simulink model "SASA_two_piezo"  (R2016a)
settings: Solver=FixedStepAuto  SolverMode=SingleTasking  StartTime=0.0  StopTime=200  FixedStep=1e-4  MaxStep=0.00001  MinStep=0.000000001  RelTol=1e-3  AbsTol=1e-3
values from neighbouring files (symbols this model uses):
  A = zeros(modes,modes)    [matrice_two_piezo.m]
  B = zeros(modes,modes)    [matrice_two_piezo.m]
  C = zeros(1,modes)    [matrice_two_piezo.m]
  c = c_num/c_den    (= -1.2195777478e-05)    [matrice_two_piezo.m]
  D = zeros(modes,modes)    [matrice_two_piezo.m]
  E = zeros(modes,modes)    [matrice_two_piezo.m]
  Q = double(Q)    [matrice_two_piezo.m]
settings Model: ExtModeTrigDuration=2  Creator=yashwanth  LastModifiedBy=yash9
settings DataIOCC: LimitDataPoints=on  SaveFormat=Array
settings OptimizationCC: OptimizeModelRefInitCode=on  MaxStackSize=64
settings DebuggingCC: SolverPrmCheckMsg=warning  AllowSymbolicDim=off
settings HardwareCC: ProdBitPerLong=64  ProdLargestAtomicFloat=None  ProdHWDeviceType=Intel->x86-64  TargetBitPerLong=64  TargetBitPerPointer=64  TargetIntDivRoundTo=Zero  TargetEndianess=LittleEndian  TargetWordSize=64  TargetHWDeviceType=Intel->x86-64
settings ModelReferenceCC: PropagateSignalLabelsOutOfModel=off
settings RTWCC: SystemTargetFile=sldrtert.tlc  TemplateMakefile=sldrtert.tmf  Description=Simulink Desktop Real-Time (ERT)  Toolchain=Arduino AVR v1.6.1  BuildConfiguration=Faster Runs  TargetLang=C++  RTWCompilerOptimization=on
settings CodeAppCC: IgnoreCustomStorageClasses=off  MaxIdLength=95
settings SimulinkDesktopRealTimeERTCC: TargetFcnLib=ansi_tfl_table_tmw.mat  TargetLibSuffix=_sldrt.lib  TargetPreCompLibLocation=C:\Program Files\MATLAB\R2016a\toolbox\sldrt\lib\win64  GenFloatMathFcnCalls=NOT IN USE  TargetLangStandard=C89/C90 (ANSI)  CodeReplacementLibrary=None  UtilityFuncGeneration=Auto  ERTMultiwordTypeDef=System defined  ERTMultiwordLength=256  MultiwordLength=2048  GenerateFullHeader=on  InferredTypesCompatibility=off  GenerateSampleERTMain=off  GenerateTestInterfaces=off  ModelReferenceCompliant=on  ParMdlRefBuildCompliant=off  CompOptLevelCompliant=on  ConcurrentExecutionCompliant=off  IncludeMdlTerminateFcn=on  GeneratePreprocessorConditionals=Use local settings  CombineOutputUpdateFcns=off  CombineSignalStateStructs=off  SuppressErrorStatus=off  ERTFirstTimeCompliant=off  IncludeFileDelimiter=Auto  ERTCustomFileBanners=off  SupportAbsoluteTime=on  LogVarNameModifier=rt_  MatFileLogging=off  MultiInstanceERTCode=off  CodeInterfacePackaging=Nonreusable function  SupportNonFinite=on  SupportComplex=on  PurelyIntegerCode=off  SupportContinuousTime=on  SupportNonInlinedSFcns=on  SupportVariableSizeSignals=off  ParenthesesLevel=Nominal  CastingMode=Nominal  MATLABClassNameForMDSCustomization=Simulink.SoftwareTarget.TargetSpecificTriggerConfigurationBase  ModelStepFunctionPrototypeControlCompliant=off  CPPClassGenCompliant=off  AutosarCompliant=off  GRTInterface=off  GenerateAllocFcn=off  UseToolchainInfoCompliant=off  GenerateSharedConstants=on  GenerateASAP2=off  InlinedParameterPlacement=Hierarchical  TargetOS=BareBoardExample  MultiInstanceErrorCode=Error  RateGroupingCode=on  RootIOFormat=Individual arguments  RTWCAPISignals=off  RTWCAPIParams=off  RTWCAPIStates=off  RTWCAPIRootIO=off  ERTSrcFileBannerTemplate=ert_code_template.cgt  ERTHdrFileBannerTemplate=ert_code_template.cgt  ERTDataSrcFileTemplate=ert_code_template.cgt  ERTDataHdrFileTemplate=ert_code_template.cgt  ERTCustomFileTemplate=example_file_process.tlc  EnableDataOwnership=off  SignalDisplayLevel=10  ParamTuneLevel=10  GlobalDataDefinition=Auto  DataDefinitionFile=global.c  GlobalDataReference=Auto  ERTFilePackagingFormat=Modular  DataReferenceFile=global.h  PreserveExpressionOrder=off  PreserveIfCondition=off  ConvertIfToSwitch=off  PreserveExternInFcnDecls=on  SuppressUnreachableDefaultCases=off  EnableSignedLeftShifts=on  EnableSignedRightShifts=on  IndentStyle=K&R  IndentSize=2  EnableUserReplacementTypes=off  MaxIdInt32=MAX_int32_T  MinIdInt32=MIN_int32_T  MaxIdUint32=MAX_uint32_T  MaxIdInt16=MAX_int16_T  MinIdInt16=MIN_int16_T  MaxIdUint16=MAX_uint16_T  MaxIdInt8=MAX_int8_T  MinIdInt8=MIN_int8_T  MaxIdUint8=MAX_uint8_T  BooleanTrueId=true  BooleanFalseId=false  MemSecPackage=--- None ---  MemSecDataConstants=Default  MemSecDataIO=Default  MemSecDataInternal=Default  MemSecDataParameters=Default  MemSecFuncInitTerm=Default  MemSecFuncExecute=Default  MemSecFuncSharedUtil=Default  CCListing=off  RebuildAll=off  ExtMode=on  ExtModeTransport=0  ExtModeStaticAlloc=off  ExtModeStaticAllocSize=1000000  ExtModeTesting=off  ExtModeMexFile=sldrtext  ExtModeIntrfLevel=Level1
settings ConfigComp: CovModelRefEnable=Off  CovSFcnEnable=off

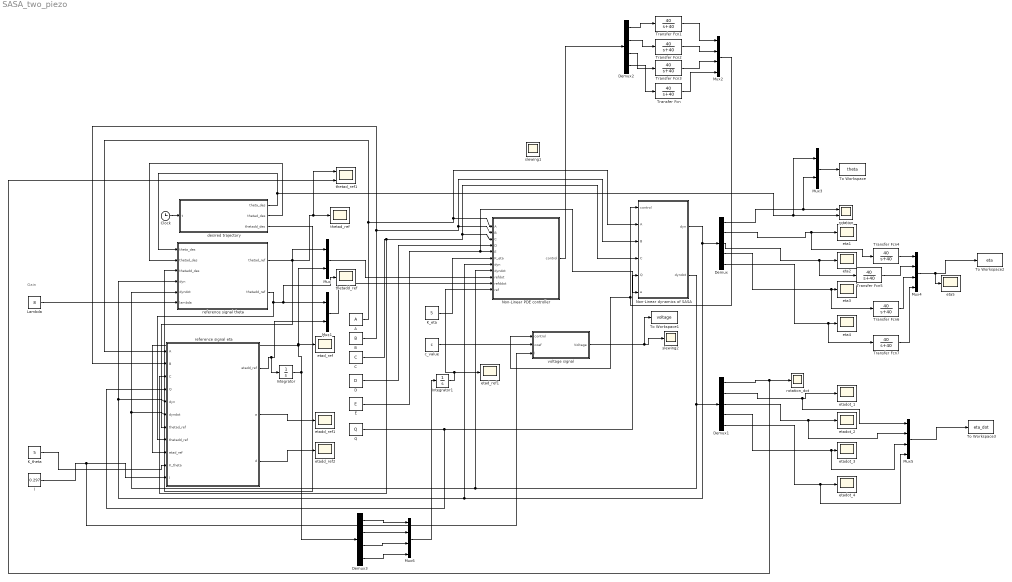
== system SASA_two_piezo ==
  note: Gain
  " Non-Linear dynamics of SASA" : Subsystem
  A : Constant  Value=A  VectorParams1D=off
  B : Constant  Value=B  VectorParams1D=off
  C : Constant  Value=C  VectorParams1D=off
  Clock : Clock
  D : Constant  Value=D  VectorParams1D=off
  Demux : Demux  Outputs=5
  Demux1 : Demux  Outputs=5
  Demux2 : Demux
  Demux3 : Demux
  E : Constant  Value=E  VectorParams1D=off
  Integrator : Integrator  InitialCondition=[0 0 0 0]
  Integrator1 : Integrator  InitialCondition=[0 0 0 0]
  K_eta : Constant  Value=5
  K_theta : Constant  Value=5
  Lambda : Constant  Value=8
  Mux : Mux  Inputs=2
  Mux1 : Mux  Inputs=2
  Mux{2,4..6} (4 alike) : Mux
  Mux3 : Mux  Inputs=2
  Non-Linear PDE controller : MATLAB Function  TreatAsAtomicUnit=on
  Q : Constant  Value=Q  VectorParams1D=off
  To Workspace : ToWorkspace  VariableName=theta  SaveFormat=Timeseries  SampleTime=-1
  To Workspace1 : ToWorkspace  VariableName=voltage  SaveFormat=Timeseries  SampleTime=-1
  To Workspace2 : ToWorkspace  VariableName=eta  SaveFormat=Timeseries  SampleTime=-1
  To Workspace3 : ToWorkspace  VariableName=eta_dot  SaveFormat=Timeseries  SampleTime=-1
  Transfer Fcn{,1..7} (8 alike) : TransferFcn  Numerator=40  Denominator=[1 40]
  c_value : Constant  Value=c
  "desired trajectory " : MATLAB Function  TreatAsAtomicUnit=on
  eta{1..5} (5 alike) : Scope
  etad_ref : Scope
  etad_ref1 : Scope
  etadd_ref1 : Scope
  etadd_ref2 : Scope
  etadot_{1..4} (4 alike) : Scope
  l : Constant  Value=0.297
  reference signal eta : MATLAB Function  TreatAsAtomicUnit=on
  reference signal theta : MATLAB Function  TreatAsAtomicUnit=on
  rotation : Scope  NumInputPorts=2
  rotation_dot : Scope
  slewing1 : Scope  NumInputPorts=2
  slewing2 : Scope
  thetad_ref : Scope
  thetad_ref1 : Scope  NumInputPorts=2
  thetadd_ref : Scope
  voltage signal : MATLAB Function  TreatAsAtomicUnit=on
  wires:
  Clock/1 -> "desired trajectory "/1(t)
  "desired trajectory "/1(theta_des) -> reference signal theta/1(theta_des), Mux3/1, rotation/2
  "desired trajectory "/2(thetad_des) -> reference signal theta/2(thetad_des)
  "desired trajectory "/3(thetadd_des) -> reference signal theta/3(thetadd_des)
  Lambda/1 -> reference signal theta/6(lambda)
  K_theta/1 -> reference signal eta/10(K_theta)
  K_eta/1 -> Non-Linear PDE controller/6(K_eta)
  " Non-Linear dynamics of SASA"/1(dyn) -> Demux/1, Non-Linear PDE controller/7(dyn), reference signal theta/4(dyn), reference signal eta/5(dyn)
  A/1 -> " Non-Linear dynamics of SASA"/2(A), Non-Linear PDE controller/1(A), reference signal eta/1(A)
  B/1 -> Non-Linear PDE controller/2(B), " Non-Linear dynamics of SASA"/3(B), reference signal eta/2(B)
  C/1 -> reference signal eta/3(C), " Non-Linear dynamics of SASA"/4(C), Non-Linear PDE controller/3(C)
  E/1 -> Non-Linear PDE controller/5(E), " Non-Linear dynamics of SASA"/6(e)
  D/1 -> Non-Linear PDE controller/4(D)
  reference signal theta/2(thetadd_ref) -> thetadd_ref/1, Mux1/1, reference signal eta/8(thetadd_ref)
  Q/1 -> reference signal eta/4(Q), " Non-Linear dynamics of SASA"/5(Q)
  l/1 -> voltage signal/3(l), reference signal eta/11(l)
  Mux/1 -> Non-Linear PDE controller/9(refdot)
  Mux1/1 -> Non-Linear PDE controller/10(refddot)
  Demux/1 -> Mux3/2, rotation/1
  c_value/1 -> voltage signal/2(coef)
  voltage signal/1(Voltage) -> To Workspace1/1, slewing2/1
  reference signal theta/1(thetad_ref) -> thetad_ref1/1, thetad_ref/1, reference signal eta/7(thetad_ref), Mux/1
  Demux/2 -> Transfer Fcn4/1, eta1/1
  Demux/3 -> Transfer Fcn5/1, eta2/1
  Demux/4 -> Transfer Fcn6/1, eta3/1
  Demux/5 -> Transfer Fcn7/1, eta4/1
  " Non-Linear dynamics of SASA"/2(dyndot) -> Demux1/1, Non-Linear PDE controller/8(dyndot), reference signal theta/5(dyndot), reference signal eta/6(dyndot)
  Demux1/1 -> thetad_ref1/2, rotation_dot/1
  reference signal eta/2(a) -> etadd_ref1/1
  reference signal eta/3(d) -> etadd_ref2/1
  Integrator/1 -> etad_ref/1, Mux/2, reference signal eta/9(etad_ref), Demux3/1
  Mux3/1 -> To Workspace/1
  Mux4/1 -> eta5/1, To Workspace2/1
  Demux1/2 -> Mux5/1, etadot_1/1
  Demux1/3 -> Mux5/2, etadot_2/1
  Demux1/4 -> Mux5/3, etadot_3/1
  Demux1/5 -> Mux5/4, etadot_4/1
  Mux5/1 -> To Workspace3/1
  Integrator1/1 -> Non-Linear PDE controller/11(ref), etad_ref1/1
  Demux3/2 -> Mux6/2
  Demux3/1 -> Mux6/1
  Demux3/3 -> Mux6/3
  Demux3/4 -> Mux6/4
  Mux6/1 -> Integrator1/1
  reference signal eta/1(etadd_ref) -> Integrator/1, Mux1/2
  Non-Linear PDE controller/1(control) -> Demux2/1
  Demux2/1 -> Transfer Fcn1/1
  Demux2/2 -> Transfer Fcn2/1
  Demux2/3 -> Transfer Fcn3/1
  Demux2/4 -> Transfer Fcn/1
  Transfer Fcn1/1 -> Mux2/1
  Transfer Fcn2/1 -> Mux2/2
  Transfer Fcn3/1 -> Mux2/3
  Transfer Fcn/1 -> Mux2/4
  Mux2/1 -> voltage signal/1(control), " Non-Linear dynamics of SASA"/1(control)
  Transfer Fcn4/1 -> Mux4/1
  Transfer Fcn5/1 -> Mux4/2
  Transfer Fcn6/1 -> Mux4/3
  Transfer Fcn7/1 -> Mux4/4

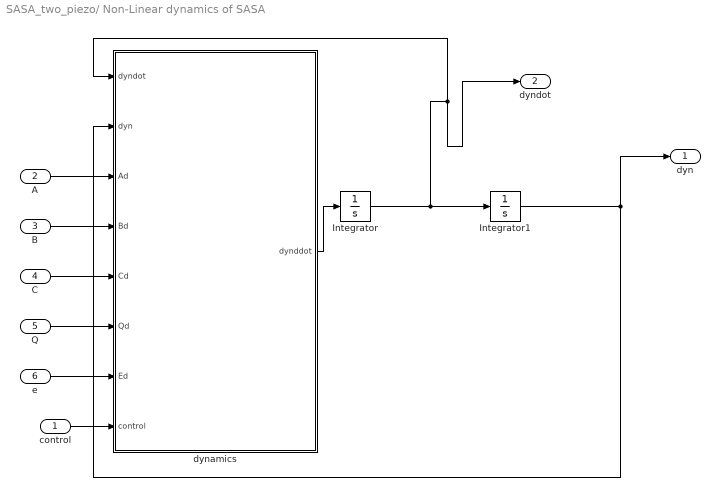
== system SASA_two_piezo/ Non-Linear dynamics of SASA ==
  control : Inport
  A : Inport  Port=2
  B : Inport  Port=3
  C : Inport  Port=4
  Q : Inport  Port=5
  e : Inport  Port=6
  Integrator : Integrator  InitialCondition=[0 0 0 0 0]  AbsoluteTolerance=1e-40
  Integrator1 : Integrator  InitialCondition=[0 0 0 0 0]
  dynamics : MATLAB Function  TreatAsAtomicUnit=on
  dyn : Outport
  dyndot : Outport  Port=2
  wires:
  control/1 -> dynamics/8(control)
  A/1 -> dynamics/3(Ad)
  B/1 -> dynamics/4(Bd)
  C/1 -> dynamics/5(Cd)
  Q/1 -> dynamics/6(Qd)
  e/1 -> dynamics/7(Ed)
  Integrator/1 -> Integrator1/1, dyndot/1, dynamics/1(dyndot)
  dynamics/1(dynddot) -> Integrator/1
  Integrator1/1 -> dyn/1, dynamics/2(dyn)

== matlab function SASA_two_piezo/desired trajectory  ==
  data: theta_des output; thetad_des output; thetadd_des output; t input
function [theta_des,thetad_des,thetadd_des] = fcn(t)

%% trajectory planned
% 
% 
% % % if t<12.5
%     
theta_des=0.001*sin(2*pi*0.02*t);
thetad_des=0.001*2*pi*0.02*cos(2*pi*0.02*t);
thetadd_des=-0.001*2*pi*2*pi*0.02*0.02*sin(2*pi*0.02*t);
% % 
% 
% theta_des=0.001*sin(2*pi*1*t);
% thetad_des=0.001*2*pi*1*cos(2*pi*1*t);
% thetadd_des=-0.001*2*pi*2*pi*sin(2*pi*1*t);
% % else
% %     
% % theta_des=0.001*sin(2*pi*0.01*t);
% % thetad_des=0.001*2*pi*0.01*cos(2*pi*0.01*t);
% % thetadd_des=-0.001*2*pi*2*pi*0.01*0.01*sin(2*pi*0.01*t);

%  theta_des=0.001;
%  thetad_des=0;
%  thetadd_des=0;
% end

% theta_des=0.005*(1-exp(-0.01*t));
% thetad_des=0.005*0.01*exp(-0.01*t);
% thetadd_des=-0.005*0.01*0.01*exp(-0.01*t);
% theta_des=(1-(1-0.5*sin(1000*t))*exp(-0.01*t));
% thetad_des=((1-0.5*sin(1000*t))*(-0.01)*exp(-0.01*t))...
%     -(0.5*1000*cos(1000*t)*exp(-0.01*t));
% thetadd_des=-(0.5*1000*cos(1000*t)*(-0.01)*exp(-0.01*t))...
%     + ((1-0.5*sin(1000*t))*0.01*0.01*exp(-0.01*t))...
%     +(0.5*1000*1000*sin(1000*t)*exp(-0.01*t))...
%     -(0.5*1000*cos(1000*t)*(-0.01)*exp(-0.01*t));


%#codegen

== matlab function SASA_two_piezo/ Non-Linear dynamics of SASA/dynamics ==
  data: dyndot input; dyn input; dynddot output; Ad input; Bd input; Cd input; Qd input; Ed input; control input
function dynddot  = fcn(dyndot,dyn,Ad,Bd,Cd,Qd,Ed,control)
%#codegen
% function dynamics of spacecraft and the rightSA
% generating matrices to use in the dynamics.
% number of modes used =4 (we use 2nd order equations here)
%dynamics of theta and eta
dyndot1=dyndot(1);
dyndot2=[dyndot(2);dyndot(3);dyndot(4);dyndot(5)];
dyn2=[dyn(2);dyn(3);dyn(4);dyn(5)];
% AA= [Qd+2*(transpose(dyn2)*(Ad-Bd)*dyn2) 2*Cd;2*Cd' 2*Ad];
% B1= [2*((dyndot1*dyndot2'*(Ad-Bd)*dyn2) + (dyn2'*(Ad-Bd)*dyndot1*dyndot2)) ;2*((-(Ad-Bd)*(dyndot1^2)*dyn2)+ (Ed*(dyn2+0.001*dyndot2)))];
% B1= [2*((dyndot1*dyndot2'*(Ad-Bd)*dyn2) + (dyn2'*(Ad-Bd)*dyndot1*dyndot2)) ;2*(-(Ad-Bd)*(dyndot1^2)*dyn2) ];
% + (Ed*(dyn2+0.001*dyndot2)
AA= [(Qd/2)+(dyn2'*(Ad-Bd)*dyn2) Cd;Cd' Ad];
B1= [(dyndot1*dyndot2'*(Ad-Bd)*dyn2) + (dyn2'*(Ad-Bd)*dyndot1*dyndot2) ;(-(Ad-Bd)*(dyndot1^2)*dyn2)+ (Ed*(dyn2+0.001*dyndot2))];
dynddot= pinv(AA)*(-B1+[0;control]);

== matlab function SASA_two_piezo/Non-Linear PDE controller ==
  data: A input; control output; B input; C input; D input; E input; K_eta input; dyn input; dyndot input; refdot input; refddot input; ref input
function control  = fcn(A,B,C,D,E,K_eta,dyn,dyndot,refdot,refddot,ref)
%% ref signals include both theta ref and eta ref
mu=0.001;
q2=[dyn(2);dyn(3);dyn(4);dyn(5)];
q1d=dyndot(1);
q2d=[dyndot(2);dyndot(3);dyndot(4);dyndot(5)];
r2d=[refdot(2);refdot(3);refdot(4);refdot(5)];
Ma=[C' A];
Ca=[-(A-B)*q1d*q2 zeros(4,4)];
%Ha= 0.0001*E*(ref +mu*r2d);
  Ha= 1*E*(q2 +mu*q2d);
Sa= K_eta*D*(q2d-r2d);
% control = - Sa ;
control = (Ma*refddot)+(Ca*refdot)+Ha- Sa;

== matlab function SASA_two_piezo/reference signal theta ==
  data: theta_des input; thetad_des input; thetadd_des input; dyn input; dyndot input; thetad_ref output; thetadd_ref output; lambda input
function [thetad_ref,thetadd_ref] = fcn(theta_des,thetad_des,thetadd_des,dyn,dyndot,lambda)
%#codegen
thetad_ref=thetad_des - lambda*(dyn(1)-theta_des);
thetadd_ref= thetadd_des - lambda*(dyndot(1)-thetad_des);

== matlab function SASA_two_piezo/reference signal eta ==
  data: etadd_ref output; A input; B input; C input; Q input; dyn input; dyndot input; thetad_ref input; thetadd_ref input; etad_ref input; K_theta input; l input; a output; d output
function [etadd_ref,a,d]= fcn(A,B,C,Q,dyn,dyndot,thetad_ref,thetadd_ref,etad_ref,K_theta,l)
%#codegen 3

q1=[dyn(2);dyn(3);dyn(4);dyn(5)];
q1d=[dyndot(2);dyndot(3);dyndot(4);dyndot(5)];
% 
% AB= A-B;
% m11= Q+ (2*q1'*(AB)*q1);
% m12= 2*C;
% c11= 2*q1d'*(AB)*q1;
% c12= 2*q1'*(AB)*dyndot(1);
% Gain =K_theta*l;
AB= A-B;
m11= (Q/2) + (q1'*(AB)*q1);
m12= C;
c11= q1d'*(AB)*q1;
c12= q1'*(AB)*dyndot(1);
Gain =K_theta*l;

%C inverse
a= - (m11*thetadd_ref);
b= -(c12*etad_ref);
c=  -(c11*thetad_ref);
d= Gain*(dyndot(1)-thetad_ref);
C_inv= pinv(m12);
etadd_ref= C_inv*(a+b+c+d);

% etadd_ref= C_inv*(a+d);

== matlab function SASA_two_piezo/voltage signal ==
  data: control input; coef input; Voltage output; l input
function Voltage = fcn(control,coef,l)

c=coef;
lb=l;
lp=7.24*10^-2; % length of the piezo
% Piezo1 location 
lp_1=1.1*10^-2; % distance of the root of the piezo from that beamroot
lp_2=lp_1+lp;

dpp=  0.47*10^-2;

lp_3= lp_2+dpp;
lp_4=lp_3+lp;



phip1_l1=(1*pi*sin(1*pi*lp_1/lb)/lb) +(((-1)^(1+1))*((1*pi/lb)^2)*lp_1);
phip2_l1= (2*pi*sin(2*pi*lp_1/lb)/lb) +(((-1)^(2+1))*((2*pi/lb)^2)*lp_1);
phip3_l1=(3*pi*sin(3*pi*lp_1/lb)/lb) +(((-1)^(3+1))*((3*pi/lb)^2)*lp_1);
phip4_l1= (4*pi*sin(4*pi*lp_1/lb)/lb) +(((-1)^(4+1))*((4*pi/lb)^2)*lp_1);

phip1_l2=(1*pi*sin(1*pi*lp_2/lb)/lb) +(((-1)^(1+1))*((1*pi/lb)^2)*lp_2);
phip2_l2= (2*pi*sin(2*pi*lp_2/lb)/lb) +(((-1)^(2+1))*((2*pi/lb)^2)*lp_2);
phip3_l2=(3*pi*sin(3*pi*lp_2/lb)/lb) +(((-1)^(3+1))*((3*pi/lb)^2)*lp_2);
phip4_l2= (4*pi*sin(4*pi*lp_2/lb)/lb) +(((-1)^(4+1))*((4*pi/lb)^2)*lp_2);



phip1_l3=(1*pi*sin(1*pi*lp_3/lb)/lb) +(((-1)^(1+1))*((1*pi/lb)^2)*lp_3);
phip2_l3= (2*pi*sin(2*pi*lp_3/lb)/lb) +(((-1)^(2+1))*((2*pi/lb)^2)*lp_3);
phip3_l3=(3*pi*sin(3*pi*lp_3/lb)/lb) +(((-1)^(3+1))*((3*pi/lb)^2)*lp_3);
phip4_l3= (4*pi*sin(4*pi*lp_3/lb)/lb) +(((-1)^(4+1))*((4*pi/lb)^2)*lp_3);

phip1_l4=(1*pi*sin(1*pi*lp_4/lb)/lb) +(((-1)^(1+1))*((1*pi/lb)^2)*lp_4);
phip2_l4= (2*pi*sin(2*pi*lp_4/lb)/lb) +(((-1)^(2+1))*((2*pi/lb)^2)*lp_4);
phip3_l4=(3*pi*sin(3*pi*lp_4/lb)/lb) +(((-1)^(3+1))*((3*pi/lb)^2)*lp_4);
phip4_l4= (4*pi*sin(4*pi*lp_4/lb)/lb) +(((-1)^(4+1))*((4*pi/lb)^2)*lp_4);

% 
% x=[phip1_l2-phip1_l1;phip2_l2-phip2_l1;phip3_l2-phip3_l1...
%     ;phip4_l2-phip4_l1];

x=[phip1_l2-phip1_l1 phip1_l4-phip1_l3;phip2_l2-phip2_l1 phip2_l4-phip2_l3;phip3_l2-phip3_l1 phip3_l4-phip3_l3...
    ;phip4_l2-phip4_l1 phip4_l4-phip4_l3];
Voltage= pinv(x'*x)*x'*control/c;
